simulink model "fdm3"  (R2020b)
settings: Solver=VariableStepAuto  StartTime=0.0  StopTime=3  RelTol=1e-3
InitFcn:
  | clear all
  | close all
  | clc
  | fs=44100;
  | ts=1/fs;
libraries: dsparch4 x13, dspvision x6
settings Model: Creator=tamim  LastModifiedBy=tamim
settings DebuggingCC: SFMachineParentedDataDiag=error

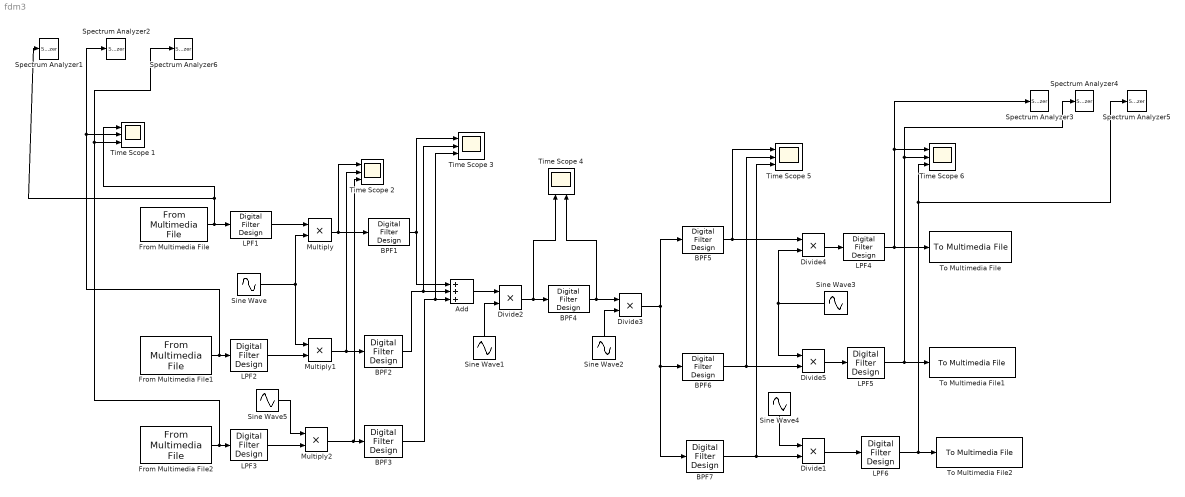
== system fdm3 ==
  Add : Sum  Inputs=+++  SampleTime=ts
  BPF{1..7} (7 alike) : dsparch4/Digital Filter Design  mwdsp_browser_bugfix_var=off
  Divide{1..5} (5 alike) : Product  Inputs=**  SampleTime=ts
  From Multimedia File : dspvision/From Multimedia File  inputFilename=F:\Level 3 Term 1\EEE310\Simulink\SSB+FDM(3 Voice)\tamim01.wav  readRange=[1 Inf]  loop=on  numPlays=inf  outputStreams=Audio only  videoDataType=single  audioDataType=double  inheritSampleTime=on  userDefinedSampleTime=1/30  noAudioOutput=off  isIntensityVideo=off  fourcc=RGB  colorVideoFormat=Separate color signals  outputEOF=off  dataOrg=Column-major  audioFrameSize=1  computeAudioFrameSize=off  outSamplingMode=Sample based
  From Multimedia File1 : dspvision/From Multimedia File  inputFilename=F:\Level 3 Term 1\EEE310\Simulink\SSB+FDM(3 Voice)\tamim02.wav  readRange=[1 Inf]  loop=on  numPlays=inf  outputStreams=Audio only  videoDataType=single  audioDataType=double  inheritSampleTime=on  userDefinedSampleTime=1/30  noAudioOutput=off  isIntensityVideo=off  fourcc=RGB  colorVideoFormat=Separate color signals  outputEOF=off  dataOrg=Column-major  audioFrameSize=1  computeAudioFrameSize=off  outSamplingMode=Sample based
  From Multimedia File2 : dspvision/From Multimedia File  inputFilename=F:\Level 3 Term 1\EEE310\Simulink\SSB+FDM(3 Voice)\tamim03.wav  readRange=[1 Inf]  loop=on  numPlays=inf  outputStreams=Audio only  videoDataType=single  audioDataType=double  inheritSampleTime=on  userDefinedSampleTime=1/30  noAudioOutput=off  isIntensityVideo=off  fourcc=RGB  colorVideoFormat=Separate color signals  outputEOF=off  dataOrg=Column-major  audioFrameSize=1  computeAudioFrameSize=off  outSamplingMode=Sample based
  LPF{1..6} (6 alike) : dsparch4/Digital Filter Design  mwdsp_browser_bugfix_var=off
  Multiply : Product  Inputs=**  SampleTime=ts
  Multiply1 : Product  Inputs=**  SampleTime=ts
  Multiply2 : Product  Inputs=**  SampleTime=ts
  Sine Wave : Sin  Frequency=2*pi*6000  SampleTime=ts
  Sine Wave1 : Sin  Frequency=2*pi*12000  SampleTime=ts
  Sine Wave2 : Sin  Frequency=2*pi*12000  SampleTime=ts
  Sine Wave3 : Sin  Frequency=2*pi*6000  SampleTime=ts
  Sine Wave4 : Sin  Frequency=2*pi*4000  SampleTime=ts
  Sine Wave5 : Sin  Frequency=2*pi*4000  SampleTime=ts
  Spectrum Analyzer{1..6} (6 alike) : SpectrumAnalyzer
  Time Scope {1..3,5..6} (5 alike) : Scope  NumInputPorts=3
  Time Scope 4 : Scope  NumInputPorts=2
  To Multimedia File : dspvision/To Multimedia File  outputFilename=F:\Level 3 Term 1\EEE310\Simulink\SSB+FDM(3 Voice)\recons1.wav  streamSelection=Audio only  videoCompressor=None (uncompressed)  audioCompressor=None (uncompressed)  imagePorts=One multidimensional signal  fileType=WAV  audioDatatype=16-bit integer  fourcc=RGB  videoQuality=75  mj2000CompFactor=10
  To Multimedia File1 : dspvision/To Multimedia File  outputFilename=F:\Level 3 Term 1\EEE310\Simulink\SSB+FDM(3 Voice)\recons2.wav  streamSelection=Audio only  videoCompressor=Lossy  audioCompressor=None (uncompressed)  imagePorts=One multidimensional signal  fileType=WAV  audioDatatype=16-bit integer  fourcc=RGB  videoQuality=75  mj2000CompFactor=10
  To Multimedia File2 : dspvision/To Multimedia File  outputFilename=F:\Level 3 Term 1\EEE310\Simulink\SSB+FDM(3 Voice)\recons3.wav  streamSelection=Audio only  videoCompressor=Lossy  audioCompressor=None (uncompressed)  imagePorts=One multidimensional signal  fileType=WAV  audioDatatype=16-bit integer  fourcc=RGB  videoQuality=75  mj2000CompFactor=10
  wires:
  BPF2/1 -> Time Scope 3/2, Add/2
  BPF1/1 -> Time Scope 3/1, Add/1
  From Multimedia File/1 -> Spectrum Analyzer1/1, Time Scope 1/1, LPF1/1
  Sine Wave/1 -> Multiply1/1, Multiply/2
  Sine Wave1/1 -> Divide2/2
  LPF5/1 -> To Multimedia File1/1, Spectrum Analyzer4/1, Time Scope 6/2
  Add/1 -> Divide2/1
  Divide2/1 -> Time Scope 4/1, BPF4/1
  Sine Wave3/1 -> Divide5/1, Divide4/2
  Divide5/1 -> LPF5/1
  BPF5/1 -> Divide4/1, Time Scope 5/1
  BPF4/1 -> Divide3/1, Time Scope 4/2
  Divide4/1 -> LPF4/1
  Multiply1/1 -> Time Scope 2/2, BPF2/1
  Multiply/1 -> BPF1/1, Time Scope 2/1
  BPF6/1 -> Time Scope 5/2, Divide5/2
  LPF1/1 -> Multiply/1
  Sine Wave2/1 -> Divide3/2
  LPF2/1 -> Multiply1/2
  From Multimedia File1/1 -> Spectrum Analyzer2/1, Time Scope 1/2, LPF2/1
  LPF4/1 -> Spectrum Analyzer3/1, Time Scope 6/1, To Multimedia File/1
  From Multimedia File2/1 -> Spectrum Analyzer6/1, Time Scope 1/3, LPF3/1
  LPF3/1 -> Multiply2/2
  Multiply2/1 -> Time Scope 2/3, BPF3/1
  BPF3/1 -> Time Scope 3/3, Add/3
  Divide3/1 -> BPF7/1, BPF6/1, BPF5/1
  Divide1/1 -> LPF6/1
  LPF6/1 -> To Multimedia File2/1, Spectrum Analyzer5/1, Time Scope 6/3
  Sine Wave4/1 -> Divide1/1
  Sine Wave5/1 -> Multiply2/1
  BPF7/1 -> Time Scope 5/3, Divide1/2
